simulink model "pendolo"  (R2024b)
settings: Solver=VariableStepAuto  StartTime=0.0  StopTime=5  MaxStep=0.001  RelTol=1e-3
values from neighbouring files (symbols this model uses):
  den_d = [1 Ts*a-1]    [pendulum_controller.m]
  K = place(A, B, desired_poles)    [pendulum_controller.m]
  num_d = [a -a]    [pendulum_controller.m]
  Ts = 0.0001    [pendulum_controller.m]
undefined symbols (not defined in the file or in its folder): dspblkCoreblockFVToolHelper, gcbh
settings Model: Creator=lorenzo  LastModifiedBy=lorenzo

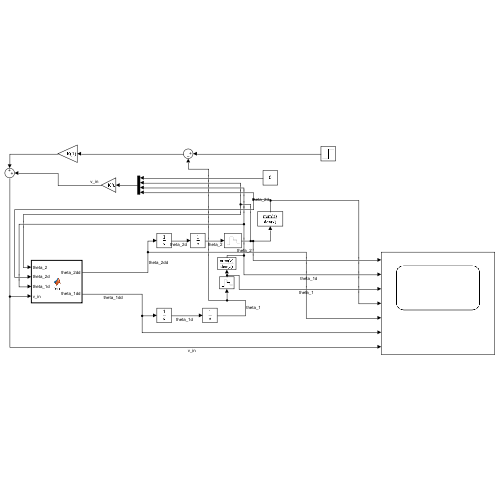
[thumbnail: Simulink's stored preview of the top-level diagram]
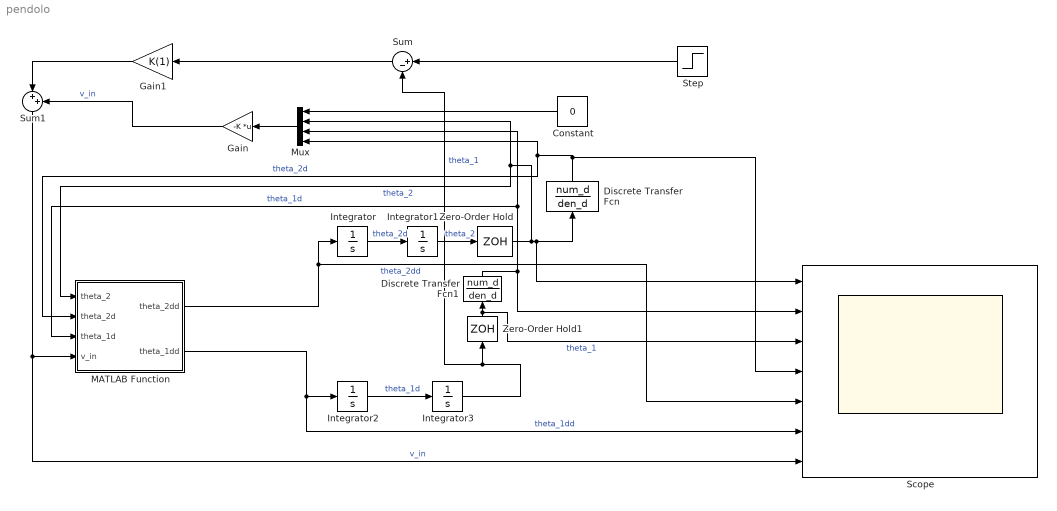
== system pendolo ==
  Constant : Constant  Value=0
  Discrete Transfer Fcn : DiscreteTransferFcn  LoadFcn=dspblkCoreblockFVToolHelper(gcbh,'load');  Numerator=num_d  Denominator=den_d
      settings: CopyFcn=dspblkCoreblockFVToolHelper(gcbh,'copy');  DeleteFcn=dspblkCoreblockFVToolHelper(gcbh,'close');  ModelCloseFcn=dspblkCoreblockFVToolHelper(gcbh,'close');  PreSaveFcn=dspblkCoreblockFVToolHelper(gcbh,'presave');  PostSaveFcn=dspblkCoreblockFVToolHelper(gcbh,'postsave');  CloseFcn=dspblkCoreblockFVToolHelper(gcbh,'close');
  Discrete Transfer Fcn1 : DiscreteTransferFcn  LoadFcn=dspblkCoreblockFVToolHelper(gcbh,'load');  Numerator=num_d  Denominator=den_d
      settings: CopyFcn=dspblkCoreblockFVToolHelper(gcbh,'copy');  DeleteFcn=dspblkCoreblockFVToolHelper(gcbh,'close');  ModelCloseFcn=dspblkCoreblockFVToolHelper(gcbh,'close');  PreSaveFcn=dspblkCoreblockFVToolHelper(gcbh,'presave');  PostSaveFcn=dspblkCoreblockFVToolHelper(gcbh,'postsave');  CloseFcn=dspblkCoreblockFVToolHelper(gcbh,'close');
  Gain : Gain  Gain=-K  Multiplication=Matrix(K*u)
  Gain1 : Gain  Gain=K(1)
  Integrator{,1..3} (4 alike) : Integrator
  MATLAB Function : MATLAB Function  TreatAsAtomicUnit=on
  Mux : Mux
  Scope : Scope  NumInputPorts=7
  Step : Step  After=pi/4  SampleTime=0
  Sum : Sum  Inputs=|+-
  Sum1 : Sum  Inputs=|++
  Zero-Order Hold : ZeroOrderHold  SampleTime=Ts
  Zero-Order Hold1 : ZeroOrderHold  SampleTime=Ts
  wires:
  MATLAB Function/1(theta_2dd) -> Integrator/1, Scope/5  "theta_2dd"
  Integrator/1 -> Integrator1/1  "theta_2d"
  Integrator1/1 -> Zero-Order Hold/1  "theta_2"
  Integrator2/1 -> Integrator3/1  "theta_1d"
  Integrator3/1 -> Zero-Order Hold1/1, Sum/2  "theta_1"
  MATLAB Function/2(theta_1dd) -> Integrator2/1, Scope/6  "theta_1dd"
  Mux/1 -> Gain/1
  Gain/1 -> Sum1/2  "v_in"
  Constant/1 -> Mux/1
  Sum/1 -> Gain1/1
  Gain1/1 -> Sum1/1
  Sum1/1 -> Scope/7, MATLAB Function/4(v_in)  "v_in"
  Discrete Transfer Fcn/1 -> MATLAB Function/2(theta_2d), Mux/4, Scope/4  "theta_2d"
  Discrete Transfer Fcn1/1 -> Scope/2, Mux/3, MATLAB Function/3(theta_1d)  "theta_1d"
  Zero-Order Hold/1 -> Discrete Transfer Fcn/1, Scope/1, MATLAB Function/1(theta_2), Mux/2  "theta_2"
  Zero-Order Hold1/1 -> Scope/3, Discrete Transfer Fcn1/1  "theta_1"
  Step/1 -> Sum/1

== matlab function pendolo/MATLAB Function ==
  data: theta_2 input; theta_2d input; theta_1d input; v_in input; theta_2dd output; theta_1dd output
function [theta_2dd,theta_1dd] = fcn(theta_2, theta_2d, theta_1d, v_in)

theta_1dd = -(0.00555*theta_1d*theta_2d*cos(theta_2)*sin(theta_2)+0.00096*theta_2d^2*sin(theta_2) ...
            -(0.00096*theta_1d^2*cos(theta_2)^2+0.02304*cos(theta_2))*sin(theta_2)+0.03641*theta_1d- ...
            0.03063*v_in)/(0.00011*cos(theta_2)^2+0.00321*sin(theta_2)^2+0.00045);
theta_2dd = -(0.00191*theta_1d*theta_2d*cos(theta_2)^2*sin(theta_2)+0.00033*theta_2d^2*cos(theta_2)*sin(theta_2) ...
            -(0.00321*theta_1d^2*cos(theta_2)+0.07752)*sin(theta_2)^3+0.01254*theta_1d*cos(theta_2) ...
            -0.01055*v_in*cos(theta_2)-(0.00044*theta_1d^2*cos(theta_2)^3+0.00053*theta_1d^2*cos(theta_2) ...
            +0.01059*cos(theta_2)^2+0.01289)*sin(theta_2))/(0.00011*cos(theta_2)^2+0.00321*sin(theta_2)^2+0.00053);
end
